simulink model "ASM1_Influentmodel1_ff"  (R2012b)
settings: Solver=ode45  StartTime=0.0  StopTime=728  RelTol=1e-5
values from neighbouring files (symbols this model uses):
  aHpercent = 75    [ASM1_Influent_init.m]    (also in ASM1_Influent_init_MC_IBU.m; ASM1_Influent_init_MC_T.m; ASM1_Influent_init_MC_TSS.m; ASM1_Influent_init_dry.m)
  Ccj_gperPEperd = 174e-3    (= 0.174)    [ASM1_Influent_init.m]    (also in ASM1_Influent_init_MC_IBU.m = RandomMatrix1(a,6); ASM1_Influent_init_MC_T.m = 2.43; ASM1_Influent_init_MC_TSS.m = 2.43; ASM1_Influent_init_dry.m)
  Ccj_HH_max = 20*Ccj_gperPEperd*PE    (= 278.4)    [ASM1_Influent_init.m]    (also in ASM1_Influent_init_MC_IBU.m = 20*Ccj_gperPEperd*PE; ASM1_Influent_init_MC_T.m = 777.6; ASM1_Influent_init_MC_TSS.m = 777.6; ASM1_Influent_init_dry.m = 55.68)
  Ccj_HH_min = 10e-6    (= 1e-05)    [ASM1_Influent_init.m]    (also in ASM1_Influent_init_MC_IBU.m; ASM1_Influent_init_MC_T.m; ASM1_Influent_init_MC_TSS.m; ASM1_Influent_init_dry.m)
  Ccj_HH_ns = 37000    [ASM1_Influent_init.m]    (also in ASM1_Influent_init_MC_IBU.m = RandomMatrix1(a,2); ASM1_Influent_init_MC_T.m; ASM1_Influent_init_MC_TSS.m; ASM1_Influent_init_dry.m)
  Ccj_HH_nv = factorM*Ccj_gperPEperd*PE    (= 27.84)    [ASM1_Influent_init.m]    (also in ASM1_Influent_init_MC_IBU.m = factorM*Ccj_gperPEperd*PE; ASM1_Influent_init_MC_T.m = 3.888; ASM1_Influent_init_MC_TSS.m = 3.888; ASM1_Influent_init_dry.m = 1.392)
  Ccj_HH_st = 1/24    (= 0.0416666666667)    [ASM1_Influent_init.m]    (also in ASM1_Influent_init_MC_IBU.m; ASM1_Influent_init_MC_T.m; ASM1_Influent_init_MC_TSS.m; ASM1_Influent_init_dry.m)
  Cli_gperPEperd = 78e-3    (= 0.078)    [ASM1_Influent_init.m]    (also in ASM1_Influent_init_MC_IBU.m = RandomMatrix1(a,5); ASM1_Influent_init_MC_T.m = 3.786; ASM1_Influent_init_MC_TSS.m = 3.786; ASM1_Influent_init_dry.m)
  Cli_HH_max = 20*Cli_gperPEperd*PE    (= 124.8)    [ASM1_Influent_init.m]    (also in ASM1_Influent_init_MC_IBU.m = 20*Cli_gperPEperd*PE; ASM1_Influent_init_MC_T.m = 1211.52; ASM1_Influent_init_MC_TSS.m = 1211.52; ASM1_Influent_init_dry.m = 24.96)
  Cli_HH_min = 10e-6    (= 1e-05)    [ASM1_Influent_init.m]    (also in ASM1_Influent_init_MC_IBU.m; ASM1_Influent_init_MC_T.m; ASM1_Influent_init_MC_TSS.m; ASM1_Influent_init_dry.m)
  Cli_HH_ns = 27000    [ASM1_Influent_init.m]    (also in ASM1_Influent_init_MC_IBU.m = RandomMatrix1(a,1); ASM1_Influent_init_MC_T.m; ASM1_Influent_init_MC_TSS.m; ASM1_Influent_init_dry.m)
  Cli_HH_nv = factorM*Cli_gperPEperd*PE    (= 12.48)    [ASM1_Influent_init.m]    (also in ASM1_Influent_init_MC_IBU.m = factorM*Cli_gperPEperd*PE; ASM1_Influent_init_MC_T.m = 6.0576; ASM1_Influent_init_MC_TSS.m = 6.0576; ASM1_Influent_init_dry.m = 0.624)
  Cli_HH_st = 1/24    (= 0.0416666666667)    [ASM1_Influent_init.m]    (also in ASM1_Influent_init_MC_IBU.m; ASM1_Influent_init_MC_T.m; ASM1_Influent_init_MC_TSS.m; ASM1_Influent_init_dry.m)
  CODpart_gperPEperd = 115.08    [ASM1_Influent_init.m]    (also in ASM1_Influent_init_MC_IBU.m; ASM1_Influent_init_MC_T.m = 80; ASM1_Influent_init_MC_TSS.m = RandomMatrix1(a,1); ASM1_Influent_init_dry.m)
  CODpart_HH_max = 20*CODpart_gperPEperd*PE    (= 184128)    [ASM1_Influent_init.m]    (also in ASM1_Influent_init_MC_IBU.m = 36825.6; ASM1_Influent_init_MC_T.m = 25600; ASM1_Influent_init_MC_TSS.m = 20*CODpart_gperPEperd*PE; ASM1_Influent_init_dry.m = 36825.6)
  CODpart_HH_min = 0.1    [ASM1_Influent_init.m]    (also in ASM1_Influent_init_MC_IBU.m; ASM1_Influent_init_MC_T.m; ASM1_Influent_init_MC_TSS.m; ASM1_Influent_init_dry.m)
  CODpart_HH_ns = 35000    [ASM1_Influent_init.m]    (also in ASM1_Influent_init_MC_IBU.m; ASM1_Influent_init_MC_T.m; ASM1_Influent_init_MC_TSS.m; ASM1_Influent_init_dry.m)
  CODpart_HH_nv = factor1*CODpart_gperPEperd*PE    (= 18412.8)    [ASM1_Influent_init.m]    (also in ASM1_Influent_init_MC_IBU.m = 3682.56; ASM1_Influent_init_MC_T.m = 2560; ASM1_Influent_init_MC_TSS.m = factor1*CODpart_gperPEperd*PE; ASM1_Influent_init_dry.m = 3682.56)
  CODpart_HH_st = 1/24    (= 0.0416666666667)    [ASM1_Influent_init.m]    (also in ASM1_Influent_init_MC_IBU.m; ASM1_Influent_init_MC_T.m; ASM1_Influent_init_MC_TSS.m; ASM1_Influent_init_dry.m)
  CODpart_Ind_kgperd = 2301.80    (= 2301.8)    [ASM1_Influent_init.m]    (also in ASM1_Influent_init_MC_IBU.m = 0; ASM1_Influent_init_MC_T.m = 0; ASM1_Influent_init_MC_TSS.m = 0; ASM1_Influent_init_dry.m)
  CODpart_Ind_max = 20*CODpart_Ind_kgperd    (= 46036)    [ASM1_Influent_init.m]    (also in ASM1_Influent_init_MC_IBU.m = 20; ASM1_Influent_init_MC_T.m = 20; ASM1_Influent_init_MC_TSS.m = 20; ASM1_Influent_init_dry.m)
  CODpart_Ind_min = 0.1    [ASM1_Influent_init.m]    (also in ASM1_Influent_init_MC_IBU.m; ASM1_Influent_init_MC_T.m; ASM1_Influent_init_MC_TSS.m; ASM1_Influent_init_dry.m)
  CODpart_Ind_ns = 21000    [ASM1_Influent_init.m]    (also in ASM1_Influent_init_MC_IBU.m; ASM1_Influent_init_MC_T.m; ASM1_Influent_init_MC_TSS.m; ASM1_Influent_init_dry.m)
  CODpart_Ind_nv = factor2*CODpart_Ind_kgperd    (= 4603.6)    [ASM1_Influent_init.m]    (also in ASM1_Influent_init_MC_IBU.m = 0; ASM1_Influent_init_MC_T.m = 0; ASM1_Influent_init_MC_TSS.m = 0; ASM1_Influent_init_dry.m)
  CODpart_Ind_st = 1/24    (= 0.0416666666667)    [ASM1_Influent_init.m]    (also in ASM1_Influent_init_MC_IBU.m; ASM1_Influent_init_MC_T.m; ASM1_Influent_init_MC_TSS.m; ASM1_Influent_init_dry.m)
  CODsol_gperPEperd = 19.31    [ASM1_Influent_init.m]    (also in ASM1_Influent_init_MC_IBU.m; ASM1_Influent_init_MC_T.m; ASM1_Influent_init_MC_TSS.m; ASM1_Influent_init_dry.m)
  CODsol_HH_max = 20*CODsol_gperPEperd*PE    (= 30896)    [ASM1_Influent_init.m]    (also in ASM1_Influent_init_MC_IBU.m = 6179.2; ASM1_Influent_init_MC_T.m = 6179.2; ASM1_Influent_init_MC_TSS.m = 6179.2; ASM1_Influent_init_dry.m = 6179.2)
  CODsol_HH_min = 0.1    [ASM1_Influent_init.m]    (also in ASM1_Influent_init_MC_IBU.m; ASM1_Influent_init_MC_T.m; ASM1_Influent_init_MC_TSS.m; ASM1_Influent_init_dry.m)
  CODsol_HH_ns = 25000    [ASM1_Influent_init.m]    (also in ASM1_Influent_init_MC_IBU.m; ASM1_Influent_init_MC_T.m; ASM1_Influent_init_MC_TSS.m; ASM1_Influent_init_dry.m)
  CODsol_HH_nv = factor1*2*CODsol_gperPEperd*PE    (= 6179.2)    [ASM1_Influent_init.m]    (also in ASM1_Influent_init_MC_IBU.m = 1235.84; ASM1_Influent_init_MC_T.m = 1235.84; ASM1_Influent_init_MC_TSS.m = 1235.84; ASM1_Influent_init_dry.m = 1235.84)
  CODsol_HH_st = 1/24    (= 0.0416666666667)    [ASM1_Influent_init.m]    (also in ASM1_Influent_init_MC_IBU.m; ASM1_Influent_init_MC_T.m; ASM1_Influent_init_MC_TSS.m; ASM1_Influent_init_dry.m)
  CODsol_Ind_kgperd = 386.24    [ASM1_Influent_init.m]    (also in ASM1_Influent_init_MC_IBU.m = 0; ASM1_Influent_init_MC_T.m = 0; ASM1_Influent_init_MC_TSS.m = 0; ASM1_Influent_init_dry.m)
  CODsol_Ind_max = 20*CODsol_Ind_kgperd    (= 7724.8)    [ASM1_Influent_init.m]    (also in ASM1_Influent_init_MC_IBU.m = 20; ASM1_Influent_init_MC_T.m = 20; ASM1_Influent_init_MC_TSS.m = 20; ASM1_Influent_init_dry.m)
  CODsol_Ind_min = 0.1    [ASM1_Influent_init.m]    (also in ASM1_Influent_init_MC_IBU.m; ASM1_Influent_init_MC_T.m; ASM1_Influent_init_MC_TSS.m; ASM1_Influent_init_dry.m)
  CODsol_Ind_ns = 11000    [ASM1_Influent_init.m]    (also in ASM1_Influent_init_MC_IBU.m; ASM1_Influent_init_MC_T.m; ASM1_Influent_init_MC_TSS.m; ASM1_Influent_init_dry.m)
  CODsol_Ind_nv = factor2*CODsol_Ind_kgperd    (= 772.48)    [ASM1_Influent_init.m]    (also in ASM1_Influent_init_MC_IBU.m = 0; ASM1_Influent_init_MC_T.m = 0; ASM1_Influent_init_MC_TSS.m = 0; ASM1_Influent_init_dry.m)
  CODsol_Ind_st = 1/24    (= 0.0416666666667)    [ASM1_Influent_init.m]    (also in ASM1_Influent_init_MC_IBU.m; ASM1_Influent_init_MC_T.m; ASM1_Influent_init_MC_TSS.m; ASM1_Influent_init_dry.m)
  Csl_gperPEperd = 0    [ASM1_Influent_init.m]    (also in ASM1_Influent_init_MC_IBU.m; ASM1_Influent_init_MC_T.m; ASM1_Influent_init_MC_TSS.m; ASM1_Influent_init_dry.m)
  Csl_HH_max = 20*Csl_gperPEperd*PE    (= 0)    [ASM1_Influent_init.m]    (also in ASM1_Influent_init_MC_IBU.m; ASM1_Influent_init_MC_T.m; ASM1_Influent_init_MC_TSS.m; ASM1_Influent_init_dry.m)
  Csl_HH_min = 0.0    (= 0)    [ASM1_Influent_init.m]    (also in ASM1_Influent_init_MC_IBU.m; ASM1_Influent_init_MC_T.m; ASM1_Influent_init_MC_TSS.m; ASM1_Influent_init_dry.m)
  Csl_HH_ns = 47000    [ASM1_Influent_init.m]    (also in ASM1_Influent_init_MC_IBU.m; ASM1_Influent_init_MC_T.m; ASM1_Influent_init_MC_TSS.m; ASM1_Influent_init_dry.m)
  Csl_HH_nv = factorM*Csl_gperPEperd*PE    (= 0)    [ASM1_Influent_init.m]    (also in ASM1_Influent_init_MC_IBU.m = factorM*Csl_gperPEperd*PE; ASM1_Influent_init_MC_T.m; ASM1_Influent_init_MC_TSS.m; ASM1_Influent_init_dry.m)
  Csl_HH_st = 1/24    (= 0.0416666666667)    [ASM1_Influent_init.m]    (also in ASM1_Influent_init_MC_IBU.m; ASM1_Influent_init_MC_T.m; ASM1_Influent_init_MC_TSS.m; ASM1_Influent_init_dry.m)
  Csl_i_gperPEperd = 0    [ASM1_Influent_init.m]    (also in ASM1_Influent_init_MC_IBU.m; ASM1_Influent_init_MC_T.m; ASM1_Influent_init_MC_TSS.m; ASM1_Influent_init_dry.m)
  Csl_i_HH_max = 20*Csl_i_gperPEperd*PE    (= 0)    [ASM1_Influent_init.m]    (also in ASM1_Influent_init_MC_IBU.m; ASM1_Influent_init_MC_T.m; ASM1_Influent_init_MC_TSS.m; ASM1_Influent_init_dry.m)
  Csl_i_HH_min = 0.0    (= 0)    [ASM1_Influent_init.m]    (also in ASM1_Influent_init_MC_IBU.m; ASM1_Influent_init_MC_T.m; ASM1_Influent_init_MC_TSS.m; ASM1_Influent_init_dry.m)
  Csl_i_HH_ns = 57000    [ASM1_Influent_init.m]    (also in ASM1_Influent_init_MC_IBU.m; ASM1_Influent_init_MC_T.m; ASM1_Influent_init_MC_TSS.m; ASM1_Influent_init_dry.m)
  Csl_i_HH_nv = factorM*Csl_i_gperPEperd*PE    (= 0)    [ASM1_Influent_init.m]    (also in ASM1_Influent_init_MC_IBU.m = factorM*Csl_i_gperPEperd*PE; ASM1_Influent_init_MC_T.m; ASM1_Influent_init_MC_TSS.m; ASM1_Influent_init_dry.m)
  Csl_i_HH_st = 1/24    (= 0.0416666666667)    [ASM1_Influent_init.m]    (also in ASM1_Influent_init_MC_IBU.m; ASM1_Influent_init_MC_T.m; ASM1_Influent_init_MC_TSS.m; ASM1_Influent_init_dry.m)
  FFfraction = 0.25    [ASM1_Influent_init.m]    (also in ASM1_Influent_init_MC_IBU.m; ASM1_Influent_init_MC_T.m = 0.4; ASM1_Influent_init_MC_TSS.m = RandomMatrix1(a,2); ASM1_Influent_init_dry.m)
  HHnoiseswitch = 1    [ASM1_Influent_init.m]    (also in ASM1_Influent_init_MC_IBU.m; ASM1_Influent_init_MC_T.m; ASM1_Influent_init_MC_TSS.m; ASM1_Influent_init_dry.m)
  HHpolnoiseswitch = 1    [ASM1_Influent_init.m]    (also in ASM1_Influent_init_MC_IBU.m; ASM1_Influent_init_MC_T.m; ASM1_Influent_init_MC_TSS.m; ASM1_Influent_init_dry.m)
  HHpopswitch = 100    [ASM1_Influent_init.m]    (also in ASM1_Influent_init_MC_IBU.m; ASM1_Influent_init_MC_T.m; ASM1_Influent_init_MC_TSS.m; ASM1_Influent_init_dry.m)
  Indnoiseswitch = 1    [ASM1_Influent_init.m]    (also in ASM1_Influent_init_MC_IBU.m; ASM1_Influent_init_MC_T.m; ASM1_Influent_init_MC_TSS.m; ASM1_Influent_init_dry.m)
  Indpolnoiseswitch = 1    [ASM1_Influent_init.m]    (also in ASM1_Influent_init_MC_IBU.m; ASM1_Influent_init_MC_T.m; ASM1_Influent_init_MC_TSS.m; ASM1_Influent_init_dry.m)
  Indpopswitch = 100    [ASM1_Influent_init.m]    (also in ASM1_Influent_init_MC_IBU.m; ASM1_Influent_init_MC_T.m = 0; ASM1_Influent_init_MC_TSS.m = 0; ASM1_Influent_init_dry.m)
  InfAmp = 1200    [ASM1_Influent_init.m]    (also in ASM1_Influent_init_MC_IBU.m; ASM1_Influent_init_MC_T.m; ASM1_Influent_init_MC_TSS.m; ASM1_Influent_init_dry.m)
  InfBias = 7100    [ASM1_Influent_init.m]    (also in ASM1_Influent_init_MC_IBU.m; ASM1_Influent_init_MC_T.m; ASM1_Influent_init_MC_TSS.m; ASM1_Influent_init_dry.m)
  Infcst = 7100    [ASM1_Influent_init.m]    (also in ASM1_Influent_init_MC_IBU.m; ASM1_Influent_init_MC_T.m; ASM1_Influent_init_MC_TSS.m; ASM1_Influent_init_dry.m)
  InfFreq = 2*pi/364    (= 0.0172614980966)    [ASM1_Influent_init.m]    (also in ASM1_Influent_init_MC_IBU.m; ASM1_Influent_init_MC_T.m; ASM1_Influent_init_MC_TSS.m; ASM1_Influent_init_dry.m)
  InfPhase = -pi*15/24    (= -1.96349540849)    [ASM1_Influent_init.m]    (also in ASM1_Influent_init_MC_IBU.m; ASM1_Influent_init_MC_T.m; ASM1_Influent_init_MC_TSS.m; ASM1_Influent_init_dry.m)
  LLrain = 3.5    [ASM1_Influent_init.m]    (also in ASM1_Influent_init_MC_IBU.m; ASM1_Influent_init_MC_T.m; ASM1_Influent_init_MC_TSS.m; ASM1_Influent_init_dry.m)
  PE = 80    [ASM1_Influent_init.m]    (also in ASM1_Influent_init_MC_IBU.m = 16; ASM1_Influent_init_MC_T.m = 16; ASM1_Influent_init_MC_TSS.m = 16; ASM1_Influent_init_dry.m = 16)
  polnoiseswitch = 1    [ASM1_Influent_init.m]    (also in ASM1_Influent_init_MC_IBU.m; ASM1_Influent_init_MC_T.m; ASM1_Influent_init_MC_TSS.m; ASM1_Influent_init_dry.m)
  Q_HH_ns = 3857    [ASM1_Influent_init.m]    (also in ASM1_Influent_init_MC_IBU.m; ASM1_Influent_init_MC_T.m; ASM1_Influent_init_MC_TSS.m; ASM1_Influent_init_dry.m)
  Q_HH_nv = 4000    [ASM1_Influent_init.m]    (also in ASM1_Influent_init_MC_IBU.m; ASM1_Influent_init_MC_T.m; ASM1_Influent_init_MC_TSS.m; ASM1_Influent_init_dry.m)
  Q_HH_st = 1/24    (= 0.0416666666667)    [ASM1_Influent_init.m]    (also in ASM1_Influent_init_MC_IBU.m; ASM1_Influent_init_MC_T.m; ASM1_Influent_init_MC_TSS.m; ASM1_Influent_init_dry.m)
  Q_Ind_ns = 2000    [ASM1_Influent_init.m]    (also in ASM1_Influent_init_MC_IBU.m; ASM1_Influent_init_MC_T.m; ASM1_Influent_init_MC_TSS.m; ASM1_Influent_init_dry.m)
  Q_Ind_nv = 15000    [ASM1_Influent_init.m]    (also in ASM1_Influent_init_MC_IBU.m; ASM1_Influent_init_MC_T.m; ASM1_Influent_init_MC_TSS.m; ASM1_Influent_init_dry.m)
  Q_Ind_st = 1/24    (= 0.0416666666667)    [ASM1_Influent_init.m]    (also in ASM1_Influent_init_MC_IBU.m; ASM1_Influent_init_MC_T.m; ASM1_Influent_init_MC_TSS.m; ASM1_Influent_init_dry.m)
  Q_SCI_ns = 1000    [ASM1_Influent_init.m]    (also in ASM1_Influent_init_MC_IBU.m; ASM1_Influent_init_MC_T.m; ASM1_Influent_init_MC_TSS.m; ASM1_Influent_init_dry.m)
  Q_SCI_nv = 0.1*InfBias    (= 710)    [ASM1_Influent_init.m]    (also in ASM1_Influent_init_MC_IBU.m; ASM1_Influent_init_MC_T.m; ASM1_Influent_init_MC_TSS.m; ASM1_Influent_init_dry.m)
  Q_SCI_st = 1    [ASM1_Influent_init.m]    (also in ASM1_Influent_init_MC_IBU.m; ASM1_Influent_init_MC_T.m; ASM1_Influent_init_MC_TSS.m; ASM1_Influent_init_dry.m)
  QHHsatmax = QperPE*50    (= 7500)    [ASM1_Influent_init.m]    (also in ASM1_Influent_init_MC_IBU.m; ASM1_Influent_init_MC_T.m; ASM1_Influent_init_MC_TSS.m; ASM1_Influent_init_dry.m)
  QHHsatmin = 0.001    [ASM1_Influent_init.m]    (also in ASM1_Influent_init_MC_IBU.m; ASM1_Influent_init_MC_T.m; ASM1_Influent_init_MC_TSS.m; ASM1_Influent_init_dry.m)
  QInd_weekday = 2500    [ASM1_Influent_init.m]    (also in ASM1_Influent_init_MC_IBU.m; ASM1_Influent_init_MC_T.m; ASM1_Influent_init_MC_TSS.m; ASM1_Influent_init_dry.m)
  QIndsatmax = QInd_weekday*10    (= 25000)    [ASM1_Influent_init.m]    (also in ASM1_Influent_init_MC_IBU.m; ASM1_Influent_init_MC_T.m; ASM1_Influent_init_MC_TSS.m; ASM1_Influent_init_dry.m)
  QIndsatmin = 0.001    [ASM1_Influent_init.m]    (also in ASM1_Influent_init_MC_IBU.m; ASM1_Influent_init_MC_T.m; ASM1_Influent_init_MC_TSS.m; ASM1_Influent_init_dry.m)
  Qpermm = 1500    [ASM1_Influent_init.m]    (also in ASM1_Influent_init_MC_IBU.m; ASM1_Influent_init_MC_T.m; ASM1_Influent_init_MC_TSS.m; ASM1_Influent_init_dry.m)
  QperPE = 150    [ASM1_Influent_init.m]    (also in ASM1_Influent_init_MC_IBU.m; ASM1_Influent_init_MC_T.m; ASM1_Influent_init_MC_TSS.m; ASM1_Influent_init_dry.m)
  QSCIsatmax = 2*(InfBias+InfAmp)    (= 16600)    [ASM1_Influent_init.m]    (also in ASM1_Influent_init_MC_IBU.m; ASM1_Influent_init_MC_T.m; ASM1_Influent_init_MC_TSS.m; ASM1_Influent_init_dry.m)
  QSCIsatmin = 0.0    (= 0)    [ASM1_Influent_init.m]    (also in ASM1_Influent_init_MC_IBU.m; ASM1_Influent_init_MC_T.m; ASM1_Influent_init_MC_TSS.m; ASM1_Influent_init_dry.m)
  rain_nm = 1    [ASM1_Influent_init.m]    (also in ASM1_Influent_init_MC_IBU.m; ASM1_Influent_init_MC_T.m; ASM1_Influent_init_MC_TSS.m; ASM1_Influent_init_dry.m)
  rain_ns = 3000    [ASM1_Influent_init.m]    (also in ASM1_Influent_init_MC_IBU.m; ASM1_Influent_init_MC_T.m; ASM1_Influent_init_MC_TSS.m; ASM1_Influent_init_dry.m)
  rain_nv = 400    [ASM1_Influent_init.m]    (also in ASM1_Influent_init_MC_IBU.m; ASM1_Influent_init_MC_T.m; ASM1_Influent_init_MC_TSS.m; ASM1_Influent_init_dry.m)
  rain_st = 1/24    (= 0.0416666666667)    [ASM1_Influent_init.m]    (also in ASM1_Influent_init_MC_IBU.m; ASM1_Influent_init_MC_T.m; ASM1_Influent_init_MC_TSS.m; ASM1_Influent_init_dry.m)
  rainmax = 1000    [ASM1_Influent_init.m]    (also in ASM1_Influent_init_MC_IBU.m; ASM1_Influent_init_MC_T.m; ASM1_Influent_init_MC_TSS.m; ASM1_Influent_init_dry.m)
  rainmin = 0    [ASM1_Influent_init.m]    (also in ASM1_Influent_init_MC_IBU.m; ASM1_Influent_init_MC_T.m; ASM1_Influent_init_MC_TSS.m; ASM1_Influent_init_dry.m)
  rainpopswitch = 100    [ASM1_Influent_init.m]    (also in ASM1_Influent_init_MC_IBU.m = 0; ASM1_Influent_init_MC_T.m = 0; ASM1_Influent_init_MC_TSS.m = 0; ASM1_Influent_init_dry.m = 0)
  SCInoiseswitch = 0    [ASM1_Influent_init.m]    (also in ASM1_Influent_init_MC_IBU.m; ASM1_Influent_init_MC_T.m; ASM1_Influent_init_MC_TSS.m; ASM1_Influent_init_dry.m)
  SCIpopswitch = 100    [ASM1_Influent_init.m]    (also in ASM1_Influent_init_MC_IBU.m; ASM1_Influent_init_MC_T.m; ASM1_Influent_init_MC_TSS.m; ASM1_Influent_init_dry.m)
  SI_max = 100*Si_in    (= 3000)    [ASM1_Influent_init.m]    (also in ASM1_Influent_init_MC_IBU.m; ASM1_Influent_init_MC_T.m; ASM1_Influent_init_MC_TSS.m; ASM1_Influent_init_dry.m)
  SI_min = 0.1    [ASM1_Influent_init.m]    (also in ASM1_Influent_init_MC_IBU.m; ASM1_Influent_init_MC_T.m; ASM1_Influent_init_MC_TSS.m; ASM1_Influent_init_dry.m)
  SI_ns = 13122    [ASM1_Influent_init.m]    (also in ASM1_Influent_init_MC_IBU.m; ASM1_Influent_init_MC_T.m; ASM1_Influent_init_MC_TSS.m; ASM1_Influent_init_dry.m)
  SI_nv = factor3*(Si_in)    (= 60)    [ASM1_Influent_init.m]    (also in ASM1_Influent_init_MC_IBU.m; ASM1_Influent_init_MC_T.m; ASM1_Influent_init_MC_TSS.m; ASM1_Influent_init_dry.m)
  SI_st = 1/24    (= 0.0416666666667)    [ASM1_Influent_init.m]    (also in ASM1_Influent_init_MC_IBU.m; ASM1_Influent_init_MC_T.m; ASM1_Influent_init_MC_TSS.m; ASM1_Influent_init_dry.m)
  SND_max = 100*Snd_in    (= 695)    [ASM1_Influent_init.m]    (also in ASM1_Influent_init_MC_IBU.m; ASM1_Influent_init_MC_T.m; ASM1_Influent_init_MC_TSS.m; ASM1_Influent_init_dry.m)
  SND_min = 0.1    [ASM1_Influent_init.m]    (also in ASM1_Influent_init_MC_IBU.m; ASM1_Influent_init_MC_T.m; ASM1_Influent_init_MC_TSS.m; ASM1_Influent_init_dry.m)
  SND_ns = 73122    [ASM1_Influent_init.m]    (also in ASM1_Influent_init_MC_IBU.m; ASM1_Influent_init_MC_T.m; ASM1_Influent_init_MC_TSS.m; ASM1_Influent_init_dry.m)
  SND_nv = factor3*(Snd_in)    (= 13.9)    [ASM1_Influent_init.m]    (also in ASM1_Influent_init_MC_IBU.m; ASM1_Influent_init_MC_T.m; ASM1_Influent_init_MC_TSS.m; ASM1_Influent_init_dry.m)
  SND_st = 1/24    (= 0.0416666666667)    [ASM1_Influent_init.m]    (also in ASM1_Influent_init_MC_IBU.m; ASM1_Influent_init_MC_T.m; ASM1_Influent_init_MC_TSS.m; ASM1_Influent_init_dry.m)
  SNH_gperPEperd = 6.89*0.85    (= 5.8565)    [ASM1_Influent_init.m]    (also in ASM1_Influent_init_MC_IBU.m = 6.36; ASM1_Influent_init_MC_T.m = 6.37; ASM1_Influent_init_MC_TSS.m = 6.37; ASM1_Influent_init_dry.m = 6.36)
  SNH_HH_max = 20*SNH_gperPEperd*PE    (= 9370.4)    [ASM1_Influent_init.m]    (also in ASM1_Influent_init_MC_IBU.m = 101760; ASM1_Influent_init_MC_T.m = 101920; ASM1_Influent_init_MC_TSS.m = 101920; ASM1_Influent_init_dry.m = 2035.2)
  SNH_HH_min = 0.1    [ASM1_Influent_init.m]    (also in ASM1_Influent_init_MC_IBU.m; ASM1_Influent_init_MC_T.m; ASM1_Influent_init_MC_TSS.m; ASM1_Influent_init_dry.m)
  SNH_HH_ns = 45000    [ASM1_Influent_init.m]    (also in ASM1_Influent_init_MC_IBU.m; ASM1_Influent_init_MC_T.m; ASM1_Influent_init_MC_TSS.m; ASM1_Influent_init_dry.m)
  SNH_HH_nv = factor1*2*SNH_gperPEperd*PE    (= 1874.08)    [ASM1_Influent_init.m]    (also in ASM1_Influent_init_MC_IBU.m = 407.04; ASM1_Influent_init_MC_T.m = 407.68; ASM1_Influent_init_MC_TSS.m = 407.68; ASM1_Influent_init_dry.m = 407.04)
  SNH_HH_st = 1/24    (= 0.0416666666667)    [ASM1_Influent_init.m]    (also in ASM1_Influent_init_MC_IBU.m; ASM1_Influent_init_MC_T.m; ASM1_Influent_init_MC_TSS.m; ASM1_Influent_init_dry.m)
  SNH_Ind_kgperd = 61.25*0.85    (= 52.0625)    [ASM1_Influent_init.m]    (also in ASM1_Influent_init_MC_IBU.m = 0; ASM1_Influent_init_MC_T.m = 0; ASM1_Influent_init_MC_TSS.m = 0; ASM1_Influent_init_dry.m)
  SNH_Ind_max = 20*SNH_Ind_kgperd    (= 1041.25)    [ASM1_Influent_init.m]    (also in ASM1_Influent_init_MC_IBU.m = 20; ASM1_Influent_init_MC_T.m = 20; ASM1_Influent_init_MC_TSS.m = 20; ASM1_Influent_init_dry.m)
  SNH_Ind_min = 0.1    [ASM1_Influent_init.m]    (also in ASM1_Influent_init_MC_IBU.m; ASM1_Influent_init_MC_T.m; ASM1_Influent_init_MC_TSS.m; ASM1_Influent_init_dry.m)
  SNH_Ind_ns = 31000    [ASM1_Influent_init.m]    (also in ASM1_Influent_init_MC_IBU.m; ASM1_Influent_init_MC_T.m; ASM1_Influent_init_MC_TSS.m; ASM1_Influent_init_dry.m)
  SNH_Ind_nv = factor2*SNH_Ind_kgperd    (= 104.125)    [ASM1_Influent_init.m]    (also in ASM1_Influent_init_MC_IBU.m = 0; ASM1_Influent_init_MC_T.m = 0; ASM1_Influent_init_MC_TSS.m = 0; ASM1_Influent_init_dry.m)
  SNH_Ind_st = 1/24    (= 0.0416666666667)    [ASM1_Influent_init.m]    (also in ASM1_Influent_init_MC_IBU.m; ASM1_Influent_init_MC_T.m; ASM1_Influent_init_MC_TSS.m; ASM1_Influent_init_dry.m)
  SNH_max = 100*Snh_in    (= 3156)    [ASM1_Influent_init.m]    (also in ASM1_Influent_init_MC_IBU.m; ASM1_Influent_init_MC_T.m; ASM1_Influent_init_MC_TSS.m; ASM1_Influent_init_dry.m)
  SNH_min = 0.1    [ASM1_Influent_init.m]    (also in ASM1_Influent_init_MC_IBU.m; ASM1_Influent_init_MC_T.m; ASM1_Influent_init_MC_TSS.m; ASM1_Influent_init_dry.m)
  SNH_ns = 63122    [ASM1_Influent_init.m]    (also in ASM1_Influent_init_MC_IBU.m; ASM1_Influent_init_MC_T.m; ASM1_Influent_init_MC_TSS.m; ASM1_Influent_init_dry.m)
  SNH_nv = factor3*(Snh_in)    (= 63.12)    [ASM1_Influent_init.m]    (also in ASM1_Influent_init_MC_IBU.m; ASM1_Influent_init_MC_T.m; ASM1_Influent_init_MC_TSS.m; ASM1_Influent_init_dry.m)
  SNH_st = 1/24    (= 0.0416666666667)    [ASM1_Influent_init.m]    (also in ASM1_Influent_init_MC_IBU.m; ASM1_Influent_init_MC_T.m; ASM1_Influent_init_MC_TSS.m; ASM1_Influent_init_dry.m)
  SS_max = 100*Ss_in    (= 6950)    [ASM1_Influent_init.m]    (also in ASM1_Influent_init_MC_IBU.m; ASM1_Influent_init_MC_T.m; ASM1_Influent_init_MC_TSS.m; ASM1_Influent_init_dry.m)
  SS_min = 0.1    [ASM1_Influent_init.m]    (also in ASM1_Influent_init_MC_IBU.m; ASM1_Influent_init_MC_T.m; ASM1_Influent_init_MC_TSS.m; ASM1_Influent_init_dry.m)
  ... (+49 more)
(part 2 of 2)

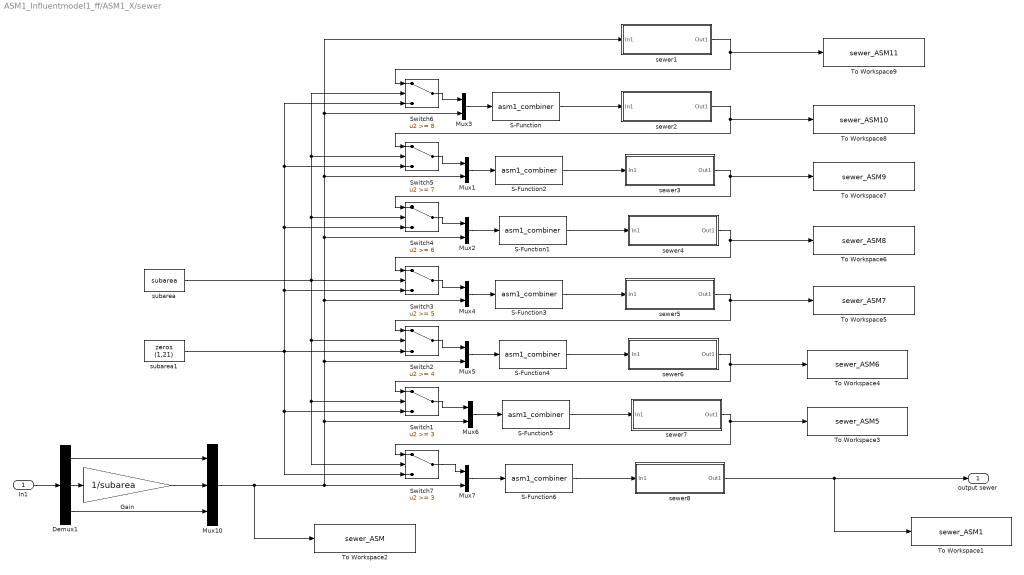
== system ASM1_Influentmodel1_ff/ASM1_X/sewer ==
  In1 : Inport
  Demux1 : Demux  Outputs=[14 1 6]
  Gain : Gain  Gain=1/subarea
  Mux{1..7} (7 alike) : Mux  Inputs=2
  Mux10 : Mux  Inputs=3
  S-Function{,1..6} (7 alike) : S-Function  FunctionName=asm1_combiner  EnableBusSupport=off
  Switch1 : Switch  Threshold=3  SaturateOnIntegerOverflow=on
  Switch2 : Switch  Threshold=4  SaturateOnIntegerOverflow=on
  Switch3 : Switch  Threshold=5  SaturateOnIntegerOverflow=on
  Switch4 : Switch  Threshold=6  SaturateOnIntegerOverflow=on
  Switch5 : Switch  Threshold=7  SaturateOnIntegerOverflow=on
  Switch6 : Switch  Threshold=8  SaturateOnIntegerOverflow=on
  Switch7 : Switch  Threshold=3  SaturateOnIntegerOverflow=on
  To Workspace1 : ToWorkspace  VariableName=sewer_ASM1  SampleTime=-1
  To Workspace2 : ToWorkspace  VariableName=sewer_ASM  SampleTime=-1
  To Workspace3 : ToWorkspace  VariableName=sewer_ASM5  SampleTime=-1
  To Workspace4 : ToWorkspace  VariableName=sewer_ASM6  SampleTime=-1
  To Workspace5 : ToWorkspace  VariableName=sewer_ASM7  SampleTime=-1
  To Workspace6 : ToWorkspace  VariableName=sewer_ASM8  SampleTime=-1
  To Workspace7 : ToWorkspace  VariableName=sewer_ASM9  SampleTime=-1
  To Workspace8 : ToWorkspace  VariableName=sewer_ASM10  SampleTime=-1
  To Workspace9 : ToWorkspace  VariableName=sewer_ASM11  SampleTime=-1
  sewer1 : Subsystem
  sewer2 : Subsystem
  sewer3 : Subsystem
  sewer4 : Subsystem
  sewer5 : Subsystem
  sewer6 : Subsystem
  sewer7 : Subsystem
  sewer8 : Subsystem
  subarea : Constant  Value=subarea
  subarea1 : Constant  Value=zeros (1,21)
  output sewer : Outport
  wires:
  In1/1 -> Demux1/1
  Demux1/2 -> Gain/1
  Demux1/1 -> Mux10/1
  Demux1/3 -> Mux10/3
  Gain/1 -> Mux10/2
  S-Function/1 -> sewer2/1(In1)
  sewer2/1(Out1) -> Switch5/1, To Workspace8/1
  S-Function2/1 -> sewer3/1(In1)
  sewer3/1(Out1) -> Switch4/1, To Workspace7/1
  S-Function1/1 -> sewer4/1(In1)
  sewer4/1(Out1) -> Switch3/1, To Workspace6/1
  S-Function3/1 -> sewer5/1(In1)
  sewer5/1(Out1) -> Switch2/1, To Workspace5/1
  sewer1/1(Out1) -> Switch6/1, To Workspace9/1
  S-Function4/1 -> sewer6/1(In1)
  sewer6/1(Out1) -> Switch1/1, To Workspace4/1
  S-Function5/1 -> sewer7/1(In1)
  sewer7/1(Out1) -> Switch7/1, To Workspace3/1
  S-Function6/1 -> sewer8/1(In1)
  Mux10/1 -> Mux1/2, Mux3/2, sewer1/1(In1), Mux2/2, Mux4/2, Mux5/2, Mux6/2, Mux7/2, To Workspace2/1
  Switch6/1 -> Mux3/1
  Mux3/1 -> S-Function/1
  Switch5/1 -> Mux1/1
  Switch4/1 -> Mux2/1
  Switch3/1 -> Mux4/1
  Switch1/1 -> Mux6/1
  Switch2/1 -> Mux5/1
  Switch7/1 -> Mux7/1
  Mux1/1 -> S-Function2/1
  Mux2/1 -> S-Function1/1
  Mux4/1 -> S-Function3/1
  Mux5/1 -> S-Function4/1
  Mux6/1 -> S-Function5/1
  Mux7/1 -> S-Function6/1
  sewer8/1(Out1) -> output sewer/1, To Workspace1/1
  subarea/1 -> Switch3/2, Switch6/2, Switch5/2, Switch4/2, Switch2/2, Switch7/2, Switch1/2
  subarea1/1 -> Switch2/3, Switch6/3, Switch5/3, Switch4/3, Switch3/3, Switch1/3, Switch7/3

== system ASM1_Influentmodel1_ff/ASM1_X/Noise application/Add noise SI ==
  In1 : Inport
  Random Number : RandomNumber  Variance=SI_nv*polnoiseswitch  Seed=SI_ns  SampleTime=SI_st
  Saturation : Saturate  UpperLimit=SI_max  LowerLimit=SI_min
  Sum : Sum  Inputs=|++  SaturateOnIntegerOverflow=on
  Out1 : Outport
  wires:
  Sum/1 -> Saturation/1
  Random Number/1 -> Sum/2
  Saturation/1 -> Out1/1
  In1/1 -> Sum/1

== system ASM1_Influentmodel1_ff/ASM1_X/Noise application/Add noise SND ==
  In1 : Inport
  Random Number : RandomNumber  Variance=SND_nv*polnoiseswitch  Seed=SND_ns  SampleTime=SND_st
  Saturation : Saturate  UpperLimit=SND_max  LowerLimit=SND_min
  Sum : Sum  Inputs=|++  SaturateOnIntegerOverflow=on
  Out1 : Outport
  wires:
  Sum/1 -> Saturation/1
  Random Number/1 -> Sum/2
  Saturation/1 -> Out1/1
  In1/1 -> Sum/1

== system ASM1_Influentmodel1_ff/ASM1_X/Noise application/Add noise SNH ==
  In1 : Inport
  Random Number : RandomNumber  Variance=SNH_nv*polnoiseswitch  Seed=SNH_ns  SampleTime=SNH_st
  Saturation : Saturate  UpperLimit=SNH_max  LowerLimit=SNH_min
  Sum : Sum  Inputs=|++  SaturateOnIntegerOverflow=on
  Out1 : Outport
  wires:
  Sum/1 -> Saturation/1
  Random Number/1 -> Sum/2
  Saturation/1 -> Out1/1
  In1/1 -> Sum/1

== system ASM1_Influentmodel1_ff/ASM1_X/Noise application/Add noise SS ==
  In1 : Inport
  Random Number : RandomNumber  Variance=SS_nv*polnoiseswitch  Seed=SS_ns  SampleTime=SS_st
  Saturation : Saturate  UpperLimit=SS_max  LowerLimit=SS_min
  Sum : Sum  Inputs=|++  SaturateOnIntegerOverflow=on
  Out1 : Outport
  wires:
  Sum/1 -> Saturation/1
  Random Number/1 -> Sum/2
  Saturation/1 -> Out1/1
  In1/1 -> Sum/1

== system ASM1_Influentmodel1_ff/ASM1_X/Noise application/Add noise XBH ==
  In1 : Inport
  Random Number : RandomNumber  Variance=XBH_nv*polnoiseswitch  Seed=XBH_ns  SampleTime=XBH_st
  Saturation : Saturate  UpperLimit=XBH_max  LowerLimit=XBH_min
  Sum : Sum  Inputs=|++  SaturateOnIntegerOverflow=on
  Out1 : Outport
  wires:
  Sum/1 -> Saturation/1
  Random Number/1 -> Sum/2
  Saturation/1 -> Out1/1
  In1/1 -> Sum/1

== system ASM1_Influentmodel1_ff/ASM1_X/Noise application/Add noise XI ==
  In1 : Inport
  Random Number : RandomNumber  Variance=XI_nv*polnoiseswitch  Seed=XI_ns  SampleTime=XI_st
  Saturation : Saturate  UpperLimit=XI_max  LowerLimit=XI_min
  Sum : Sum  Inputs=|++  SaturateOnIntegerOverflow=on
  Out1 : Outport
  wires:
  Sum/1 -> Saturation/1
  Random Number/1 -> Sum/2
  Saturation/1 -> Out1/1
  In1/1 -> Sum/1

== system ASM1_Influentmodel1_ff/ASM1_X/Noise application/Add noise XND ==
  In1 : Inport
  Random Number : RandomNumber  Variance=XND_nv*polnoiseswitch  Seed=XND_ns  SampleTime=XND_st
  Saturation : Saturate  UpperLimit=XND_max  LowerLimit=XND_min
  Sum : Sum  Inputs=|++  SaturateOnIntegerOverflow=on
  Out1 : Outport
  wires:
  Sum/1 -> Saturation/1
  Random Number/1 -> Sum/2
  Saturation/1 -> Out1/1
  In1/1 -> Sum/1

== system ASM1_Influentmodel1_ff/ASM1_X/Noise application/Add noise XS ==
  In1 : Inport
  Random Number : RandomNumber  Variance=XS_nv*polnoiseswitch  Seed=XS_ns  SampleTime=XS_st
  Saturation : Saturate  UpperLimit=XS_max  LowerLimit=XS_min
  Sum : Sum  Inputs=|++  SaturateOnIntegerOverflow=on
  Out1 : Outport
  wires:
  Sum/1 -> Saturation/1
  Random Number/1 -> Sum/2
  Saturation/1 -> Out1/1
  In1/1 -> Sum/1

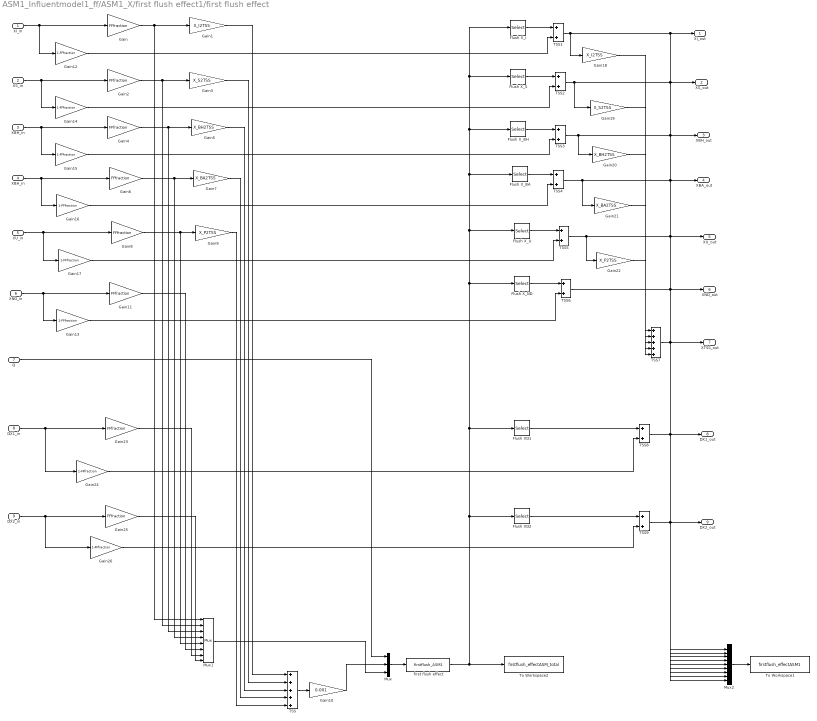
== system ASM1_Influentmodel1_ff/ASM1_X/first flush effect1/first flush effect ==
  XI_in : Inport
  XS_in : Inport  Port=2
  XBH_in : Inport  Port=3
  XBA_in : Inport  Port=4
  XU_in : Inport  Port=5
  XND_in : Inport  Port=6
  Q : Inport  Port=7
  DX1_in : Inport  Port=8
  DX2_in : Inport  Port=9
  Flush XD1 : Selector  InputPortWidth=19  IndexOptions=Index vector (dialog)  Indices=[9]  OutputSizes=1
  Flush XD2 : Selector  InputPortWidth=19  IndexOptions=Index vector (dialog)  Indices=[10]  OutputSizes=1
  Flush X_BA : Selector  InputPortWidth=19  IndexOptions=Index vector (dialog)  Indices=[6]  OutputSizes=1
  Flush X_BH : Selector  InputPortWidth=19  IndexOptions=Index vector (dialog)  Indices=[5]  OutputSizes=1
  Flush X_I : Selector  InputPortWidth=19  IndexOptions=Index vector (dialog)  Indices=[3]  OutputSizes=1
  Flush X_ND : Selector  InputPortWidth=19  IndexOptions=Index vector (dialog)  Indices=[8]  OutputSizes=1
  Flush X_S : Selector  InputPortWidth=19  IndexOptions=Index vector (dialog)  Indices=[4]  OutputSizes=1
  Flush X_U : Selector  InputPortWidth=19  IndexOptions=Index vector (dialog)  Indices=[7]  OutputSizes=1
  Gain{,2,4,6,8,11,23,25} (8 alike) : Gain  Gain=FFfraction
  Gain1 : Gain  Gain=X_I2TSS
  Gain10 : Gain  Gain=0.001
  Gain{12..17,24,26} (8 alike) : Gain  Gain=1-FFfraction
  Gain18 : Gain  Gain=X_I2TSS
  Gain19 : Gain  Gain=X_S2TSS
  Gain20 : Gain  Gain=X_BH2TSS
  Gain21 : Gain  Gain=X_BA2TSS
  Gain22 : Gain  Gain=X_P2TSS
  Gain3 : Gain  Gain=X_S2TSS
  Gain5 : Gain  Gain=X_BH2TSS
  Gain7 : Gain  Gain=X_BA2TSS
  Gain9 : Gain  Gain=X_P2TSS
  Mux : Mux  Inputs=3
  Mux1 : Mux  Inputs=8
  Mux2 : Mux  Inputs=9
  TSS : Sum  Inputs=+++++
  TSS{1..6,8..9} (8 alike) : Sum
  TSS7 : Sum  Inputs=+++++
  To Workspace1 : ToWorkspace  VariableName=firstflush_effectASM1  SampleTime=-1
  To Workspace2 : ToWorkspace  VariableName=firstflush_effectASM_total  SampleTime=-1
  first flush effect : S-Function  FunctionName=firstflush_ASM1  Parameters=ASM1_XINIT, SSPARS  EnableBusSupport=off
  XI_out : Outport
  XS_out : Outport  Port=2
  XBH_out : Outport  Port=3
  XBA_out : Outport  Port=4
  XU_out : Outport  Port=5
  XND_out : Outport  Port=6
  XTSS_out : Outport  Port=7
  DX1_out : Outport  Port=8
  DX2_out : Outport  Port=9
  wires:
  XI_in/1 -> Gain/1, Gain12/1
  Gain/1 -> Gain1/1, Mux1/1
  XS_in/1 -> Gain2/1, Gain14/1
  Gain2/1 -> Gain3/1, Mux1/2
  XBH_in/1 -> Gain4/1, Gain15/1
  Gain4/1 -> Gain5/1, Mux1/3
  XBA_in/1 -> Gain6/1, Gain16/1
  Gain6/1 -> Gain7/1, Mux1/4
  XU_in/1 -> Gain8/1, Gain17/1
  Gain8/1 -> Gain9/1, Mux1/5
  Gain11/1 -> Mux1/6
  XND_in/1 -> Gain11/1, Gain13/1
  Gain12/1 -> TSS1/2
  Flush X_I/1 -> TSS1/1
  Flush X_S/1 -> TSS2/1
  Gain14/1 -> TSS2/2
  Flush X_BH/1 -> TSS3/1
  Gain15/1 -> TSS3/2
  Gain16/1 -> TSS4/2
  Flush X_BA/1 -> TSS4/1
  Gain17/1 -> TSS5/2
  Flush X_U/1 -> TSS5/1
  Gain13/1 -> TSS6/2
  Flush X_ND/1 -> TSS6/1
  TSS1/1 -> Gain18/1, XI_out/1, Mux2/1
  TSS2/1 -> Gain19/1, XS_out/1, Mux2/2
  TSS3/1 -> Gain20/1, XBH_out/1, Mux2/3
  TSS4/1 -> Gain21/1, XBA_out/1, Mux2/4
  TSS5/1 -> Gain22/1, XU_out/1, Mux2/5
  TSS6/1 -> XND_out/1, Mux2/6
  Gain18/1 -> TSS7/1
  Gain19/1 -> TSS7/2
  Gain20/1 -> TSS7/3
  Gain21/1 -> TSS7/4
  Gain22/1 -> TSS7/5
  TSS7/1 -> XTSS_out/1, Mux2/7
  Mux2/1 -> To Workspace1/1
  DX1_in/1 -> Gain23/1, Gain24/1
  DX2_in/1 -> Gain25/1, Gain26/1
  Gain1/1 -> TSS/1
  Gain3/1 -> TSS/2
  Gain5/1 -> TSS/3
  Gain7/1 -> TSS/4
  Gain9/1 -> TSS/5
  Mux1/1 -> Mux/3
  Q/1 -> Mux/1
  Mux/1 -> first flush effect/1
  TSS/1 -> Gain10/1
  Gain10/1 -> Mux/2
  first flush effect/1 -> Flush X_I/1, Flush X_S/1, Flush X_BH/1, Flush X_BA/1, Flush X_U/1, Flush X_ND/1, Flush XD1/1, Flush XD2/1, To Workspace2/1
  Gain24/1 -> TSS8/2
  TSS8/1 -> DX1_out/1, Mux2/8
  Gain26/1 -> TSS9/2
  TSS9/1 -> DX2_out/1, Mux2/9
  Gain23/1 -> Mux1/7
  Gain25/1 -> Mux1/8
  Flush XD2/1 -> TSS9/1
  Flush XD1/1 -> TSS8/1

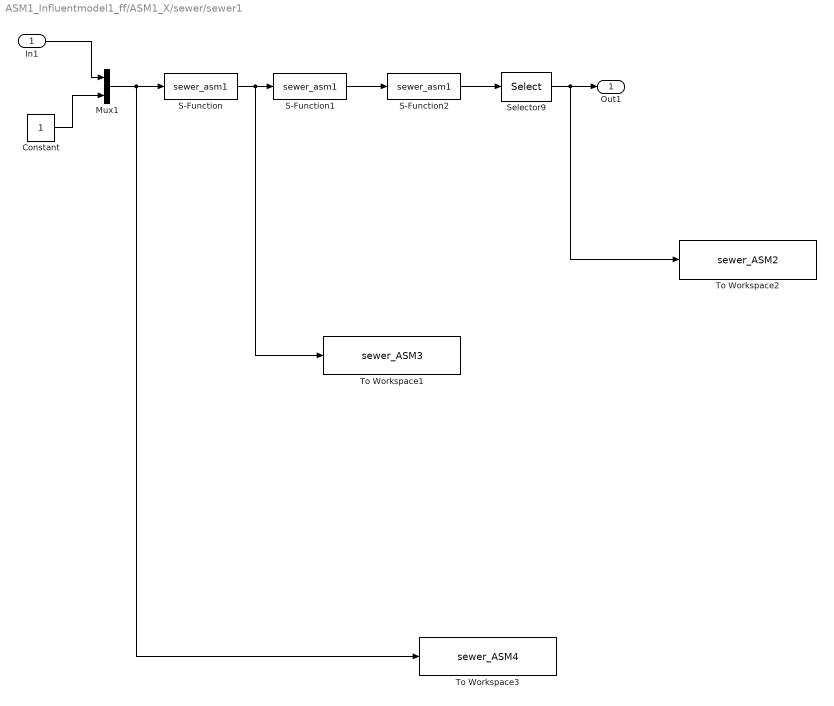
== system ASM1_Influentmodel1_ff/ASM1_X/sewer/sewer1 ==
  In1 : Inport
  Constant : Constant
  Mux1 : Mux  Inputs=2
  S-Function : S-Function  FunctionName=sewer_asm1  Parameters=ASM1_SEWERINIT, ASM1_PARS, SPAR, SOSAT, ASMX, KLa  EnableBusSupport=off
  S-Function1 : S-Function  FunctionName=sewer_asm1  Parameters=ASM1_SEWERINIT, ASM1_PARS, SPAR, SOSAT, ASMX, KLa  EnableBusSupport=off
  S-Function2 : S-Function  FunctionName=sewer_asm1  Parameters=ASM1_SEWERINIT, ASM1_PARS, SPAR, SOSAT, ASMX, KLa  EnableBusSupport=off
  Selector9 : Selector  InputPortWidth=22  IndexOptions=Index vector (dialog)  Indices=[1 2 3 4 5 6 7 8 9 10 11 12 13 14 15 16 17 18 19 20 21]  OutputSizes=1
  To Workspace1 : ToWorkspace  VariableName=sewer_ASM3  SampleTime=-1
  To Workspace2 : ToWorkspace  VariableName=sewer_ASM2  SampleTime=-1
  To Workspace3 : ToWorkspace  VariableName=sewer_ASM4  SampleTime=-1
  Out1 : Outport
  wires:
  S-Function/1 -> S-Function1/1, To Workspace1/1
  S-Function1/1 -> S-Function2/1
  S-Function2/1 -> Selector9/1
  Mux1/1 -> S-Function/1, To Workspace3/1
  Constant/1 -> Mux1/2
  In1/1 -> Mux1/1
  Selector9/1 -> Out1/1, To Workspace2/1

== system ASM1_Influentmodel1_ff/ASM1_X/sewer/sewer2 ==
  In1 : Inport
  Constant : Constant
  Mux1 : Mux  Inputs=2
  S-Function : S-Function  FunctionName=sewer_asm1  Parameters=ASM1_SEWERINIT, ASM1_PARS, SPAR, SOSAT, ASMX, KLa  EnableBusSupport=off
  S-Function1 : S-Function  FunctionName=sewer_asm1  Parameters=ASM1_SEWERINIT, ASM1_PARS, SPAR, SOSAT, ASMX, KLa  EnableBusSupport=off
  S-Function2 : S-Function  FunctionName=sewer_asm1  Parameters=ASM1_SEWERINIT, ASM1_PARS, SPAR, SOSAT, ASMX, KLa  EnableBusSupport=off
  Selector9 : Selector  InputPortWidth=22  IndexOptions=Index vector (dialog)  Indices=[1 2 3 4 5 6 7 8 9 10 11 12 13 14 15 16 17 18 19 20 21]  OutputSizes=1
  Out1 : Outport
  wires:
  Constant/1 -> Mux1/2
  Selector9/1 -> Out1/1
  In1/1 -> Mux1/1
  S-Function/1 -> S-Function1/1
  S-Function1/1 -> S-Function2/1
  Mux1/1 -> S-Function/1
  S-Function2/1 -> Selector9/1

== system ASM1_Influentmodel1_ff/ASM1_X/sewer/sewer3 ==
  In1 : Inport
  Constant : Constant
  Mux1 : Mux  Inputs=2
  S-Function : S-Function  FunctionName=sewer_asm1  Parameters=ASM1_SEWERINIT, ASM1_PARS, SPAR, SOSAT, ASMX, KLa  EnableBusSupport=off
  S-Function1 : S-Function  FunctionName=sewer_asm1  Parameters=ASM1_SEWERINIT, ASM1_PARS, SPAR, SOSAT, ASMX, KLa  EnableBusSupport=off
  S-Function2 : S-Function  FunctionName=sewer_asm1  Parameters=ASM1_SEWERINIT, ASM1_PARS, SPAR, SOSAT, ASMX, KLa  EnableBusSupport=off
  Selector9 : Selector  InputPortWidth=22  IndexOptions=Index vector (dialog)  Indices=[1 2 3 4 5 6 7 8 9 10 11 12 13 14 15 16 17 18 19 20 21]  OutputSizes=1
  Out1 : Outport
  wires:
  Constant/1 -> Mux1/2
  In1/1 -> Mux1/1
  Selector9/1 -> Out1/1
  S-Function/1 -> S-Function1/1
  S-Function1/1 -> S-Function2/1
  S-Function2/1 -> Selector9/1
  Mux1/1 -> S-Function/1

== system ASM1_Influentmodel1_ff/ASM1_X/sewer/sewer4 ==
  In1 : Inport
  Constant : Constant
  Mux1 : Mux  Inputs=2
  S-Function : S-Function  FunctionName=sewer_asm1  Parameters=ASM1_SEWERINIT, ASM1_PARS, SPAR, SOSAT, ASMX, KLa  EnableBusSupport=off
  S-Function1 : S-Function  FunctionName=sewer_asm1  Parameters=ASM1_SEWERINIT, ASM1_PARS, SPAR, SOSAT, ASMX, KLa  EnableBusSupport=off
  S-Function2 : S-Function  FunctionName=sewer_asm1  Parameters=ASM1_SEWERINIT, ASM1_PARS, SPAR, SOSAT, ASMX, KLa  EnableBusSupport=off
  Selector9 : Selector  InputPortWidth=22  IndexOptions=Index vector (dialog)  Indices=[1 2 3 4 5 6 7 8 9 10 11 12 13 14 15 16 17 18 19 20 21]  OutputSizes=1
  Out1 : Outport
  wires:
  Constant/1 -> Mux1/2
  In1/1 -> Mux1/1
  Selector9/1 -> Out1/1
  S-Function/1 -> S-Function1/1
  S-Function1/1 -> S-Function2/1
  S-Function2/1 -> Selector9/1
  Mux1/1 -> S-Function/1

== system ASM1_Influentmodel1_ff/ASM1_X/sewer/sewer5 ==
  In1 : Inport
  Constant : Constant
  Mux1 : Mux  Inputs=2
  S-Function : S-Function  FunctionName=sewer_asm1  Parameters=ASM1_SEWERINIT, ASM1_PARS, SPAR, SOSAT, ASMX, KLa  EnableBusSupport=off
  S-Function1 : S-Function  FunctionName=sewer_asm1  Parameters=ASM1_SEWERINIT, ASM1_PARS, SPAR, SOSAT, ASMX, KLa  EnableBusSupport=off
  S-Function2 : S-Function  FunctionName=sewer_asm1  Parameters=ASM1_SEWERINIT, ASM1_PARS, SPAR, SOSAT, ASMX, KLa  EnableBusSupport=off
  Selector9 : Selector  InputPortWidth=22  IndexOptions=Index vector (dialog)  Indices=[1 2 3 4 5 6 7 8 9 10 11 12 13 14 15 16 17 18 19 20 21]  OutputSizes=1
  Out1 : Outport
  wires:
  Constant/1 -> Mux1/2
  In1/1 -> Mux1/1
  Selector9/1 -> Out1/1
  S-Function/1 -> S-Function1/1
  S-Function1/1 -> S-Function2/1
  S-Function2/1 -> Selector9/1
  Mux1/1 -> S-Function/1

== system ASM1_Influentmodel1_ff/ASM1_X/sewer/sewer6 ==
  In1 : Inport
  Constant : Constant
  Mux1 : Mux  Inputs=2
  S-Function : S-Function  FunctionName=sewer_asm1  Parameters=ASM1_SEWERINIT, ASM1_PARS, SPAR, SOSAT, ASMX, KLa  EnableBusSupport=off
  S-Function1 : S-Function  FunctionName=sewer_asm1  Parameters=ASM1_SEWERINIT, ASM1_PARS, SPAR, SOSAT, ASMX, KLa  EnableBusSupport=off
  S-Function2 : S-Function  FunctionName=sewer_asm1  Parameters=ASM1_SEWERINIT, ASM1_PARS, SPAR, SOSAT, ASMX, KLa  EnableBusSupport=off
  Selector9 : Selector  InputPortWidth=22  IndexOptions=Index vector (dialog)  Indices=[1 2 3 4 5 6 7 8 9 10 11 12 13 14 15 16 17 18 19 20 21]  OutputSizes=1
  Out1 : Outport
  wires:
  Constant/1 -> Mux1/2
  In1/1 -> Mux1/1
  Selector9/1 -> Out1/1
  S-Function/1 -> S-Function1/1
  S-Function1/1 -> S-Function2/1
  S-Function2/1 -> Selector9/1
  Mux1/1 -> S-Function/1

== system ASM1_Influentmodel1_ff/ASM1_X/sewer/sewer7 ==
  In1 : Inport
  Constant : Constant
  Mux1 : Mux  Inputs=2
  S-Function : S-Function  FunctionName=sewer_asm1  Parameters=ASM1_SEWERINIT, ASM1_PARS, SPAR, SOSAT, ASMX, KLa  EnableBusSupport=off
  S-Function1 : S-Function  FunctionName=sewer_asm1  Parameters=ASM1_SEWERINIT, ASM1_PARS, SPAR, SOSAT, ASMX, KLa  EnableBusSupport=off
  S-Function2 : S-Function  FunctionName=sewer_asm1  Parameters=ASM1_SEWERINIT, ASM1_PARS, SPAR, SOSAT, ASMX, KLa  EnableBusSupport=off
  Selector9 : Selector  InputPortWidth=22  IndexOptions=Index vector (dialog)  Indices=[1 2 3 4 5 6 7 8 9 10 11 12 13 14 15 16 17 18 19 20 21]  OutputSizes=1
  Out1 : Outport
  wires:
  Constant/1 -> Mux1/2
  In1/1 -> Mux1/1
  Selector9/1 -> Out1/1
  S-Function/1 -> S-Function1/1
  S-Function1/1 -> S-Function2/1
  S-Function2/1 -> Selector9/1
  Mux1/1 -> S-Function/1

== system ASM1_Influentmodel1_ff/ASM1_X/sewer/sewer8 ==
  In1 : Inport
  Constant : Constant
  Mux1 : Mux  Inputs=2
  S-Function : S-Function  FunctionName=sewer_asm1  Parameters=ASM1_SEWERINIT, ASM1_PARS, SPAR, SOSAT, ASMX, KLa  EnableBusSupport=off
  S-Function1 : S-Function  FunctionName=sewer_asm1  Parameters=ASM1_SEWERINIT, ASM1_PARS, SPAR, SOSAT, ASMX, KLa  EnableBusSupport=off
  S-Function2 : S-Function  FunctionName=sewer_asm1  Parameters=ASM1_SEWERINIT, ASM1_PARS, SPAR, SOSAT, ASMX, KLa  EnableBusSupport=off
  Selector9 : Selector  InputPortWidth=22  IndexOptions=Index vector (dialog)  Indices=[1 2 3 4 5 6 7 8 9 10 11 12 13 14 15 16 17 18 19 20 21 ]  OutputSizes=1
  Out1 : Outport
  wires:
  Constant/1 -> Mux1/2
  In1/1 -> Mux1/1
  Selector9/1 -> Out1/1
  S-Function/1 -> S-Function1/1
  S-Function1/1 -> S-Function2/1
  S-Function2/1 -> Selector9/1
  Mux1/1 -> S-Function/1
